simulink model "dcmotors"  (R2018a)
settings: Solver=VariableStepAuto  StartTime=0.0  StopTime=10.0  RelTol=1e-3
libraries: arduinolib x2
settings Model: SimulationMode=external  Creator=stevengong  LastModifiedBy=stevengong

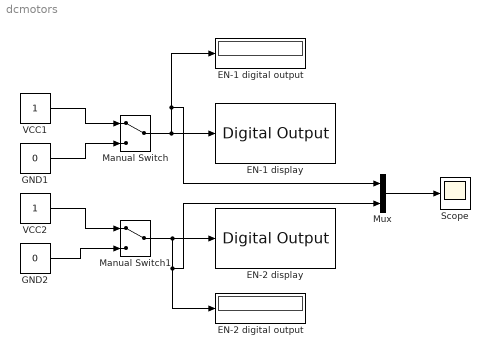
== system dcmotors ==
  EN-1 digital output : Display
  EN-1 display : arduinolib/Digital Output  pinNumber=5  blockPlatform=arduino
  "EN-2 digital output " : Display
  EN-2 display : arduinolib/Digital Output  pinNumber=6  blockPlatform=arduino
  GND1 : Constant  Value=0
  GND2 : Constant  Value=0
  Manual Switch : ManualSwitch
  Manual Switch1 : ManualSwitch
  Mux : Mux  Inputs=2
  Scope : Scope
  VCC1 : Constant
  VCC2 : Constant
  wires:
  VCC2/1 -> Manual Switch1/1
  GND2/1 -> Manual Switch1/2
  GND1/1 -> Manual Switch/2
  VCC1/1 -> Manual Switch/1
  Manual Switch/1 -> Mux/1, EN-1 digital output/1, EN-1 display/1
  Manual Switch1/1 -> Mux/2, "EN-2 digital output "/1, EN-2 display/1
  Mux/1 -> Scope/1
